simulink library "libEngineThrustLookUpTables"  (R2020b)
settings: Solver=VariableStepAuto  StartTime=0.0  StopTime=10.0  RelTol=1e-3
undefined symbols (not defined in the file): data
settings Model: Creator=caatay  LastModifiedBy=caatay

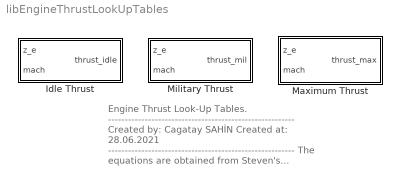
== system libEngineThrustLookUpTables ==
  note: Engine Thrust Look-Up Tables.
      | --------------------------------------------------------
      | Created by: Cagatay SAHİN
      | Created at: 28.06.2021
      | --------------------------------------------------------
      | The equations are obtained from
      | Steven's textbook.
      | The reference book can be found in
      | "references folder".
      | --------------------------------------------------------
      | for question:
      | cagataysahin44@gmail.com
  Idle Thrust : Subsystem  mask(Engine Model - Look-Up Tables - Idle Thrust Engine Data){data=data}
      mask prompts: data "Engine Look-Up Table Data"
      mask help: Aircraft's Engine Idle Thrust 2-D Look-Up Tables with atmospheric parameters and altitude information.
      mask Help:
      | This block is used for obtain idle thrust with using interpolation method on 2-D look-up tables.
      | --------------------------------------------------------------------------------------------------------------------------------------------------
      | Input of the function:
      | 	mach: Mach number.
      | 	z_e: Altitude (ft)
      | Output of the function:
      | 	idleThrust: Idle Thrust value (lbf)
      | --------------------------------------------------------------------------------------------------------------------------------------------------
      | All equations can be found in Steven's text book. Reference can be found in "literature" subfolder.
      | for question: "cagataysahin44@gmail.com"
      mask Display:
      | port_label('input',1,'z_{e}','texmode','on');
      | port_label('input',2,'M','texmode','on');
      | 
      | port_label('output',1,'T_{idle}','texmode','on');
  Maximum Thrust : Subsystem  mask(Engine Model - Look-Up Tables - Maximum Thrust Engine Data){data=data}
      mask prompts: data "Engine Look-up Table Data"
      mask help: Aircraft's Engine Maximum Thrust 2-D Look-Up Tables with atmospheric parameters and altitude information.
      mask Help:
      | This block is used for obtain maxşmum thrust with using interpolation method on 2-D look-up tables.
      | --------------------------------------------------------------------------------------------------------------------------------------------------
      | Input of the function:
      | 	mach: Mach number.
      | 	z_e: Altitude (ft)
      | Output of the function:
      | 	idleThrust: Maximum Thrust value (lbf)
      | --------------------------------------------------------------------------------------------------------------------------------------------------
      | All equations can be found in Steven's text book. Reference can be found in "literature" subfolder.
      | for question: "cagataysahin44@gmail.com"
      mask Display:
      | port_label('input',1,'z_{e}','texmode','on');
      | port_label('input',2,'M','texmode','on');
      | 
      | port_label('output',1,'T_{max}','texmode','on');
  Military Thrust : Subsystem  mask(Engine Model - Look-Up Tables - Military Thrust Engine Data){data=data}
      mask prompts: data "Engine Look-up Table Data"
      mask help: Aircraft's Engine Military Thrust 2-D Look-Up Tables with atmospheric parameters and altitude information.
      mask Help:
      | This block is used for obtain military thrust with using interpolation method on 2-D look-up tables.
      | --------------------------------------------------------------------------------------------------------------------------------------------------
      | Input of the function:
      | 	mach: Mach number.
      | 	z_e: Altitude (ft)
      | Output of the function:
      | 	idleThrust: Military Thrust value (lbf)
      | --------------------------------------------------------------------------------------------------------------------------------------------------
      | All equations can be found in Steven's text book. Reference can be found in "literature" subfolder.
      | for question: "cagataysahin44@gmail.com"
      mask Display:
      | port_label('input',1,'z_{e}','texmode','on');
      | port_label('input',2,'M','texmode','on');
      | 
      | port_label('output',1,'T_{mil}','texmode','on');

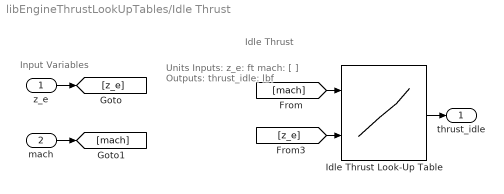
== system libEngineThrustLookUpTables/Idle Thrust ==
  note: Idle Thrust
  note: Units
      | Inputs:
      | z_e: ft
      | mach: [ ]
      | Outputs:
      | thrust_idle: lbf
  note: Input Variables
  z_e : Inport
  mach : Inport  Port=2
  Idle Thrust Look-Up Table : Lookup_n-D  BreakpointsForDimension1=data.engine.thrust.table.refSignals.mach  BreakpointsForDimension2=data.engine.thrust.table.refSignals.z_e  Table=data.engine.thrust.table.idle.T  InternalRulePriority=Speed  RndMeth=Simplest  InputSameDT=on
      settings: InputPortMap=u0,u1
  thrust_idle : Outport  VectorParamsAs1DForOutWhenUnconnected=off
  wires:
  [z_e] -> Idle Thrust Look-Up Table/2
  z_e/1 -> [z_e]
  Idle Thrust Look-Up Table/1 -> thrust_idle/1
  mach/1 -> [mach]
  [mach] -> Idle Thrust Look-Up Table/1

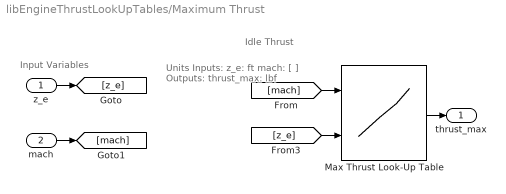
== system libEngineThrustLookUpTables/Maximum Thrust ==
  note: Idle Thrust
  note: Units
      | Inputs:
      | z_e: ft
      | mach: [ ]
      | Outputs:
      | thrust_max: lbf
  note: Input Variables
  z_e : Inport
  mach : Inport  Port=2
  Max Thrust Look-Up Table : Lookup_n-D  BreakpointsForDimension1=data.engine.thrust.table.refSignals.mach  BreakpointsForDimension2=data.engine.thrust.table.refSignals.z_e  Table=data.engine.thrust.table.maximum.T  InternalRulePriority=Speed  RndMeth=Simplest  InputSameDT=on
      settings: InputPortMap=u0,u1
  thrust_max : Outport  VectorParamsAs1DForOutWhenUnconnected=off
  wires:
  [z_e] -> Max Thrust Look-Up Table/2
  z_e/1 -> [z_e]
  Max Thrust Look-Up Table/1 -> thrust_max/1
  mach/1 -> [mach]
  [mach] -> Max Thrust Look-Up Table/1

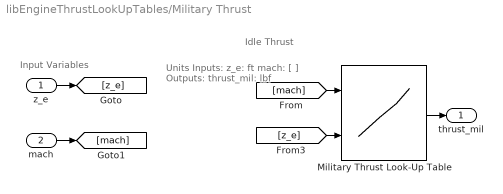
== system libEngineThrustLookUpTables/Military Thrust ==
  note: Idle Thrust
  note: Units
      | Inputs:
      | z_e: ft
      | mach: [ ]
      | Outputs:
      | thrust_mil: lbf
  note: Input Variables
  z_e : Inport
  mach : Inport  Port=2
  Military Thrust Look-Up Table : Lookup_n-D  BreakpointsForDimension1=data.engine.thrust.table.refSignals.mach  BreakpointsForDimension2=data.engine.thrust.table.refSignals.z_e  Table=data.engine.thrust.table.military.T  InternalRulePriority=Speed  RndMeth=Simplest  InputSameDT=on
      settings: InputPortMap=u0,u1
  thrust_mil : Outport  VectorParamsAs1DForOutWhenUnconnected=off
  wires:
  [z_e] -> Military Thrust Look-Up Table/2
  z_e/1 -> [z_e]
  Military Thrust Look-Up Table/1 -> thrust_mil/1
  mach/1 -> [mach]
  [mach] -> Military Thrust Look-Up Table/1
